simulink model "MPC_JUB27"  (R2020b)
settings: Solver=FixedStepDiscrete  StartTime=0.0  StopTime=StopTime  FixedStep=Ts  MaxStep=0.01  RelTol=1e-3
values from neighbouring files (symbols this model uses):
  dumax = [0.1; 1]    [CarregaDados.m]    (also in casadi_block_Control.m = evalin('base','dumax'))
  dumin = [0 ; 0]    [CarregaDados.m]    (also in casadi_block_Control.m = evalin('base','dumin'))
  f_buscaLimites_sym = evalin('base', 'f_buscaLimites_sym')    [casadi_block_Control.m]
  FreqAlvoIni = 55    [CarregaDados.m]
  Hc = 2    [CarregaDadosMPC.m]    (also in casadi_block_Control.m = evalin('base','Hc'))
  Hp = 5    [CarregaDadosMPC.m]    (also in casadi_block_Control.m = evalin('base','Hp'))
  LimiteProporcao = Ts/TempoESN    (= 641.025641026)    [CarregaDados.m]
  NumCasasDecimais = 1    [CarregaDados.m]
  PassoMPC = 3    [CarregaDadosMPC.m]
  Plano = readtable('PlanoAceleracaoErro.xlsx')    [CarregaDados.m]
  PMonAlvoIni = LimitaFaixa(PMonAlvoIni,FaixaPChegada)    [CarregaDados.m]
  Qu = diag([1  1])    [CarregaDadosMPC.m]    (also in casadi_block_Control.m = evalin('base','Qu'))
  Qy = diag([1  1])    [CarregaDadosMPC.m]    (also in casadi_block_Control.m = evalin('base','Qy'))
  R = [1  1]    [CarregaDadosMPC.m]    (also in casadi_block_Control.m = diag(repmat(R,1,Hc)))
  Rede_Processo = load('weightsESNx_TR300_TVaz0.8_RaioE0.1.mat')    [CarregaDados.m]
  SNR = 20    [CarregaDados.m]
  Ts = 10    [CarregaDados.m]
  UIni = repmat(UIni,Hc,1)    [casadi_block_Control.m]
  umax = [FreqMaxMin(1); PMonAlvoMaxMin(1)]    [CarregaDados.m]    (also in casadi_block_Control.m = evalin('base','umax'))
  umin = [FreqMaxMin(2); PMonAlvoMaxMin(2)]    [CarregaDados.m]    (also in casadi_block_Control.m = evalin('base','umin'))
  UsaPlano = 1    [CarregaDados.m]
  XIni = repmat(XIni,1+Hp,1)    [casadi_block_Control.m]
undefined symbols (not defined in the file or in its folder): awgn, BTP, Interpola, MatrizSimulador, MatrizSimuladorContas, TabelaIsometricas
libraries: simulink x1
settings Model: Creator=odilo  LastModifiedBy=leize
settings SolverCC: AlgebraicLoopSolver=LineSearch
settings DebuggingCC: InheritedTsInSrcMsg=none

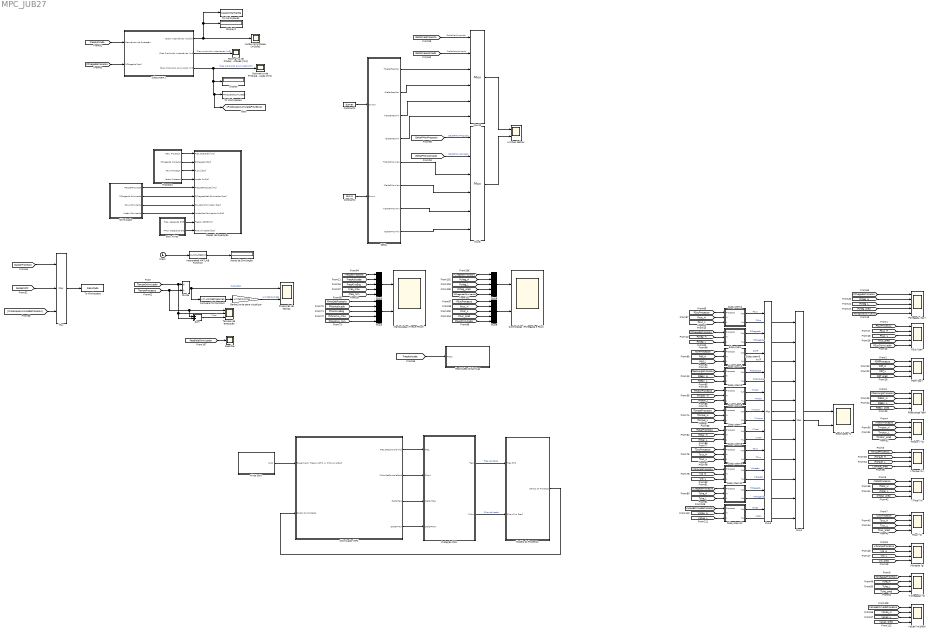
== system MPC_JUB27 ==
  Alvos ENG : Subsystem
  Clock : Clock
  Compare To Constant : simulink/Logic and Bit Operations/Compare To Constant  relop=<=  const=LimiteProporcao  OutDataTypeStr=boolean
  Constant1 : Constant  Value=dumax
  Constant2 : Constant  Value=dumin
  Controladas (PChegada e PSuc) : Scope  NumInputPorts=2
  Delta : Subsystem
  Display : Display
  Display3 : Display
  Divide : Product  Inputs=*/
  ENG. Alvos : Subsystem
  Estimativa de Produção Acumulada [m3] : Scope
  Estimativa de Produção instantânea [m3] : Scope
  Feasible : Scope
  GanhoLimite para visualizar : Gain  Gain=LimiteProporcao
  Horas de Simulação : Display
  I.Torque (A) : Scope  NumInputPorts=4
  I.Total (A) : Scope  NumInputPorts=4
  Interpreted MATLAB Function : MATLABFcn  MATLABFcn=round(u/3600,2)
  Limites DeltaU : Scope  NumInputPorts=2
  Manipuladas (Freq e PMon) : Scope  NumInputPorts=2
  Mapas de Operação : Subsystem  mask{PlotaMapas=1, HabilitaRastro=1, Tsim=MatrizSimulador, TsimContas=MatrizSimuladorContas, BTP=BTP, TabelaIsometricas=TabelaIsometricas, FreqIni=UIni(1), PChegadaIni=XIni(2), PSucIni=XIni(1), VazaoIni=XIni(11), FreqAlvoIni=FreqAlvoIni, PMonAlvoIni=PMonAlvoIni}
      mask prompts: PlotaMapas "Plotar Mapas (1/0)?"; HabilitaRastro "Habilita Rastro do Plot (1/0)?"; Tsim "Matriz do Simulador"; TsimContas "Matriz do Simulador para Limites"; BTP "Matriz BTP"; TabelaIsometricas "Tabela Curvas Isometricas"; FreqIni "Frequencia Inicial [Hz]"; PChegadaIni "PChegada Inicial [bar]"; PSucIni "PSuc Inicial [bar]"; VazaoIni "Vazao Inicial [m3/d]"; FreqAlvoIni "Frequencia ALVO Inicial [Hz]"; PMonAlvoIni "PChegada ALVO [bar]"
      mask DialogControl DescTextVar Prompt: MAPAS DE OPERAÇÃO
      mask DialogControl ParameterGroupVar Prompt: Tabelas Petrobras e configurações dos Mapas de Operação
      mask DialogControl ParameterGroupVar_copy Prompt: Dados do Processo
      mask DialogControl ParameterGroupVar_copy_copy_copy Prompt: Dados Engenharia (Alvos)
  Modelo do Processo : Subsystem  mask{ESN=Rede_Processo, YIni=XIni, UIni=UIni, SNR=SNR, NumCasasDecimais=NumCasasDecimais, MatrizSimulador=MatrizSimulador}
      mask prompts: ESN "Estruturada ESN"; YIni "Condicoes iniciais das variaveis"; UIni "Condicao Inicial das manipuladas (Freq e PMon)"; SNR "Relação Sinal Ruido aplicada"; NumCasasDecimais "Numero de casas decimais"; MatrizSimulador "Matriz do Simulador Petrobras"
  Mux : Mux  Inputs=3
  Mux{1..2,8..9} (4 alike) : Mux  Inputs=5
  Mux10 : Mux  Inputs=6
  Mux3 : Mux  Inputs=11
  Mux4 : Mux  Inputs=11
  Mux6 : Mux  Inputs=6
  Otimizador : Subsystem
  Otimizador MPC : Subsystem  mask{umax=umax, umin=umin, dumax=dumax, dumin=dumin, Hp=Hp, Hc=Hc, Qy=Qy, R=R, Qu=Qu, PassoMPC=PassoMPC}
      mask prompts: umax "Max valores para as manipuladas [Freq ;  PMonAlvo]"; umin "Min valores para as manipuladas [Freq ;  PMonAlvo]"; dumax "Max passo [Freq ;  PMonAlvo]"; dumin "Min passo [Freq ;  PMonAlvo]"; Hp "Horizonte de Predicao"; Hc "Horizonte de Controle"; Qy "Peso das Controladas [PSuc ; PChegada]"; R "Peso das Manipuladas [Freq ;  PMonAlvo]"; Qu "Peso dos alvos [Freq ;  PMonAlvo]"; PassoMPC "Passos para o controle atuar"
      mask DialogControl UserParameters Prompt: PARAMETROS DO USUARIO
      mask DialogControl ControlParameters Prompt: PARAMETROS DO CONTROLADOR
  PChegada (bar) : Scope  NumInputPorts=5
  PDescarga (bar) : Scope  NumInputPorts=4
  PDiff (bar) : Scope  NumInputPorts=4
  PSuc (bar) : Scope  NumInputPorts=5
  Processo : Subsystem
  Proporção de Tempo : Scope  NumInputPorts=2
  Proteção MPA : Subsystem  mask{DesabilitaMPA=0, DeltaUmax=dumax}
      mask prompts: DesabilitaMPA "Desabilita MPA"; DeltaUmax "Delta U Maximo (Freq e PMon)"
  Restrições % : Scope  NumInputPorts=2
  Restrições Dinâmicas : Subsystem
  Subsystem : Subsystem
  Subsystem1 : Subsystem  mask{MatrizSimulador=MatrizSimulador, DeltaT=Ts, QIni=XIni(11)}
      mask prompts: MatrizSimulador "Matriz do Simulador Petrobras"; DeltaT "Periodo de amostragem (s)"; QIni "Vazao Inicial (m3/dia)"
  Subsystem10 : Subsystem
  Subsystem12 : Subsystem
  Subsystem2 : Subsystem
  Subsystem3 : Subsystem
  Subsystem4 : Subsystem
  Subsystem5 : Subsystem
  Subsystem6 : Subsystem
  Subsystem7 : Subsystem
  Subsystem8 : Subsystem
  Subsystem9 : Subsystem
  Sum : Sum
  T.Chegada(°C) : Scope  NumInputPorts=4
  TMotor (°C) : Scope  NumInputPorts=4
  TSuc(°C) : Scope  NumInputPorts=4
  Tempos de execução : Scope  NumInputPorts=3
  To Workspace : ToWorkspace  VariableName=Resultado  SampleTime=-1
  To Workspace1 : ToWorkspace  VariableName=ProducaoAcumulada  SaveFormat=Timeseries  SampleTime=-1
  To Workspace2 : ToWorkspace  VariableName=VazaoInstantanea  SaveFormat=Timeseries  SampleTime=-1
  Vazão (m3/dia) : Scope  NumInputPorts=4
  Vazão Instantânea [m3/dia] : Scope
  Vibração (g) : Scope  NumInputPorts=4
  wires:
  [TempoProcesso] -> Sum/1, Tempos de execução/1, Divide/2
  [ITotalProcesso] -> I.Total (A)/1
  [TMotorProcesso] -> TMotor (°C)/1
  [VibracaoProcesso] -> Vibração (g)/1
  [TSucProcesso] -> TSuc(°C)/1
  [PDiffProcesso] -> PDiff (bar)/1
  [PDescargaProcesso] -> PDescarga (bar)/1
  [PSucProcesso] -> PSuc (bar)/1
  [Freq_max] -> Mux1/4
  [Freq_min] -> Mux1/5
  [FreqAlvoEng] -> Mux1/3
  [Psuc_H] -> PSuc (bar)/2
  [Psuc_L] -> PSuc (bar)/3
  [Pdif_H] -> PDiff (bar)/2
  [Pdif_L] -> PDiff (bar)/3
  [Pdif_pred] -> PDiff (bar)/4
  [Pdesc_H] -> PDescarga (bar)/2
  [Pdesc_L] -> PDescarga (bar)/3
  [Pdesc_pred] -> PDescarga (bar)/4
  [Tmotor_H] -> TMotor (°C)/2
  [Tmotor_L] -> TMotor (°C)/3
  [Tmotor_pred] -> TMotor (°C)/4
  [ITorqueProcesso] -> I.Torque (A)/1
  [ITorque_H] -> I.Torque (A)/2
  [ITorque_L] -> I.Torque (A)/3
  [Ctorque_pred] -> I.Torque (A)/4
  [ITotal_H] -> I.Total (A)/2
  [ITotal_L] -> I.Total (A)/3
  [CTotal_pred] -> I.Total (A)/4
  [Tsuc_H] -> TSuc(°C)/2
  [Tsuc_L] -> TSuc(°C)/3
  [Tsuc_pred] -> TSuc(°C)/4
  [Vib_H] -> Vibração (g)/2
  [Vib_L] -> Vibração (g)/3
  [Vib_pred] -> Vibração (g)/4
  [TChegadaProcesso] -> T.Chegada(°C)/1
  [Tche_H] -> T.Chegada(°C)/2
  [Tche_L] -> T.Chegada(°C)/3
  [Tche_pred] -> T.Chegada(°C)/4
  [SaidasMPC] -> Mux/2
  Mux/1 -> To Workspace/1
  [DadosProcesso] -> Mux/1
  Otimizador MPC/2(PMonSetControle[bar]) -> Proteção MPA/2(PMon.)
  [FreqAplicada] -> Mux1/2
  [Psuc_pred] -> PSuc (bar)/4
  [PSucOtimizador] -> PSuc (bar)/5
  [PChegadaProcesso] -> PChegada (bar)/1
  [Pcheg_H] -> PChegada (bar)/2
  [Pcheg_L] -> PChegada (bar)/3
  [Pcheg_pred] -> PChegada (bar)/4
  [PChegadaOtimizador] -> PChegada (bar)/5
  [TempoOtimizador] -> Sum/2, Tempos de execução/2, Divide/1
  Otimizador MPC/1(Freq.SetControle [Hz]) -> Proteção MPA/1(Freq.)
  [FreqAplicada] -> Subsystem1/1(Frequência de Operação)
  [PChegadaProcesso] -> Subsystem1/2(PChegada [bar])
  Subsystem1/2("Óleo Produzido Instantâneo (m3) ") -> Estimativa de Produção instantânea [m3]/1  "Óleo produzido Instantâneo (m3)"
  Subsystem1/3(Óleo Produzido Acumulado (m3)) -> [ProducaoAcumuladaProcesso], To Workspace1/1, Display/1, Estimativa de Produção Acumulada [m3]/1  "Óleo produzido acumulado(m3)"
  Subsystem1/1(Vazão Instantânea (m3/dia)) -> To Workspace2/1, Display3/1, Vazão Instantânea [m3/dia]/1
  Sum/1 -> Tempos de execução/3  "Total"
  Mux1/1 -> Manipuladas (Freq e PMon)/1
  [PMonAlvo_min] -> Mux2/5
  [PMonAlvo_max] -> Mux2/4
  [PMonAplicado] -> Mux2/2
  Mux2/1 -> Manipuladas (Freq e PMon)/2
  [PChegadaProcesso] -> Subsystem/1(Processo)
  [Pcheg_H] -> Subsystem/2(H)
  [Pcheg_L] -> Subsystem/3(L)
  [PSucProcesso] -> Subsystem2/1(Processo)
  [Psuc_H] -> Subsystem2/2(H)
  [Psuc_L] -> Subsystem2/3(L)
  [PDiffProcesso] -> Subsystem3/1(Processo)
  [Pdif_H] -> Subsystem3/2(H)
  [Pdif_L] -> Subsystem3/3(L)
  [PDescargaProcesso] -> Subsystem4/1(Processo)
  [Pdesc_H] -> Subsystem4/2(H)
  [Pdesc_L] -> Subsystem4/3(L)
  [Tmotor_L] -> Subsystem5/3(L)
  [Tmotor_H] -> Subsystem5/2(H)
  [TMotorProcesso] -> Subsystem5/1(Processo)
  [ITorqueProcesso] -> Subsystem6/1(Processo)
  [ITorque_H] -> Subsystem6/2(H)
  [ITorque_L] -> Subsystem6/3(L)
  [ITotalProcesso] -> Subsystem7/1(Processo)
  [ITotal_H] -> Subsystem7/2(H)
  [ITotal_L] -> Subsystem7/3(L)
  [TSucProcesso] -> Subsystem8/1(Processo)
  [Tsuc_H] -> Subsystem8/2(H)
  [Tsuc_L] -> Subsystem8/3(L)
  [VibracaoProcesso] -> Subsystem9/1(Processo)
  [Vib_H] -> Subsystem9/2(H)
  [Vib_L] -> Subsystem9/3(L)
  [TChegadaProcesso] -> Subsystem10/1(Processo)
  [Tche_H] -> Subsystem10/2(H)
  [Tche_L] -> Subsystem10/3(L)
  Mux3/1 -> Restrições %/1
  Mux4/1 -> Restrições %/2
  Subsystem/2(%L) -> Mux4/2  "PChegada"
  Subsystem2/2(%L) -> Mux4/1  "PSuc"
  Subsystem/1(%H) -> Mux3/2  "PChegada"
  Subsystem2/1(%H) -> Mux3/1  "PSuc"
  Subsystem3/1(%H) -> Mux3/3  "PDiff"
  Subsystem3/2(%L) -> Mux4/3  "PDiff"
  Subsystem4/1(%H) -> Mux3/4  "PDescarga"
  Subsystem4/2(%L) -> Mux4/4  "PDescarga"
  Subsystem5/2(%L) -> Mux4/5  "TMotor"
  Subsystem5/1(%H) -> Mux3/5  "TMotor"
  Subsystem6/2(%L) -> Mux4/6  "I.Torque"
  Subsystem6/1(%H) -> Mux3/6  "I.Torque"
  Subsystem7/2(%L) -> Mux4/7  "I.Total"
  Subsystem7/1(%H) -> Mux3/7  "I.Total"
  Subsystem8/2(%L) -> Mux4/8  "TSuc"
  Subsystem8/1(%H) -> Mux3/8  "TSuc"
  Subsystem9/2(%L) -> Mux4/9  "Vibração"
  Mux10/1 -> Limites DeltaU/1
  Constant1/1 -> Delta/1(dumax)
  Constant2/1 -> Delta/2(dumin)
  Delta/2(-DeltaFreqMax) -> Mux10/4
  Delta/3(+DeltaFreqMin) -> Mux10/5
  Delta/4(-DeltaFreqMin) -> Mux10/6
  Mux6/1 -> Limites DeltaU/2
  Clock/1 -> Interpreted MATLAB Function/1
  Interpreted MATLAB Function/1 -> Horas de Simulação/1
  [DeltaPMonProposto] -> Mux6/1  "DeltaPMonProposto"
  Delta/5(+DeltaPMonMax) -> Mux6/3
  Delta/6(-DeltaPMonMax) -> Mux6/4
  Delta/7(+DeltaPMonMin) -> Mux6/5
  Delta/8(-DeltaPMonMin) -> Mux6/6
  [PChegadaOtimizador] -> Mux8/5
  [Pcheg_pred] -> Mux8/4
  [Pcheg_L] -> Mux8/3
  [Pcheg_H] -> Mux8/2
  [PChegadaProcesso] -> Mux8/1
  [PSucOtimizador] -> Mux9/5
  [Psuc_pred] -> Mux9/4
  [Psuc_L] -> Mux9/3
  [Psuc_H] -> Mux9/2
  [PSucProcesso] -> Mux9/1
  Mux9/1 -> Controladas (PChegada e PSuc)/2
  Mux8/1 -> Controladas (PChegada e PSuc)/1
  [FeadibleOtimizador] -> Feasible/1
  Processo/1(Freq. Processo) -> Mapas de Operação/1(Freq.Operação [Hz])
  Processo/2(PChegada Processo) -> Mapas de Operação/2(PChegada [bar])
  Otimizador/2(PChegada Otimizador) -> Mapas de Operação/6(PChegadaSet Otimizador [bar])
  Otimizador/3(PSuc Otimizador) -> Mapas de Operação/7(PSucSet Otimizador [bar])
  ENG. Alvos/1(Freq. desejada ENG) -> Mapas de Operação/9(FreqAlvoENG[Hz])
  ENG. Alvos/2(PMon Desejada ENG) -> Mapas de Operação/10(PMonAlvoENG [bar])
  Processo/3(PSuc Processo) -> Mapas de Operação/3(P.Suc [bar])
  [DeltaFreqProposto] -> Mux10/1  "DeltaFreqProposto"
  [DeltaFreqAplicado] -> Mux10/2  "DeltaFreqAplicado"
  Delta/1(+DeltaFreqMax) -> Mux10/3
  [DeltaPMonAplicado] -> Mux6/2  "DeltaPMonAplicado"
  Proteção MPA/1(Freq) -> Modelo do Processo/1(Freq [Hz])  "Freq.Aplicada"
  Otimizador MPC/3(DeltaFreq) -> Proteção MPA/3(Delta Freq.)
  Otimizador MPC/4(DeltaPMon) -> Proteção MPA/4(DeltaPMon)
  Proteção MPA/2(PMon) -> Modelo do Processo/2(PMonAlvo [bar])  "PMonAplicada"
  [FreqSetProposta] -> Mux1/1
  [PMonSetProposto] -> Mux2/1
  Otimizador/1(FreqSetProposta) -> Mapas de Operação/5(FreqSetProposta [Hz])
  [PMonAlvoEng] -> Mux2/3
  [Vazao_L] -> Vazão (m3/dia)/3
  [Vazao_H] -> Vazão (m3/dia)/2
  [VazaoEstimadaProcesso] -> Vazão (m3/dia)/1
  [VazaoEstimadaProcesso] -> Subsystem12/1(Processo)
  [Vazao_H] -> Subsystem12/2(H)
  [Vazao_L] -> Subsystem12/3(L)
  Subsystem12/1(%H) -> Mux3/11  "Vazao"
  Subsystem12/2(%L) -> Mux4/11  "Vazao"
  Subsystem10/2(%L) -> Mux4/10  "TChegada"
  Subsystem9/1(%H) -> Mux3/9  "Vibração"
  Subsystem10/1(%H) -> Mux3/10  "TChegada"
  [Vazao_pred] -> Vazão (m3/dia)/4
  Modelo do Processo/1(Dados do Processo) -> Otimizador MPC/2(Dados do Processo)
  [ProducaoAcumuladaProcesso] -> Mux/3
  Divide/1 -> Proporção de Tempo/1, Compare To Constant/1  "Proporção"
  Compare To Constant/1 -> GanhoLimite para visualizar/1
  GanhoLimite para visualizar/1 -> Proporção de Tempo/2  "LimiteProporção"
  Processo/4(Vazão Processo) -> Mapas de Operação/4(Vazão [m3/d])
  Otimizador/4(Vazão Otimizador) -> Mapas de Operação/8(VazãoSet Otimizador [m3/d])
  Alvos ENG/1(Out1) -> Otimizador MPC/1(Engenharia: FreqAlvo[Hz]  e  PMonAlvo[bar])
  [FreqAplicada] -> Restrições Dinâmicas/1(Freq1)

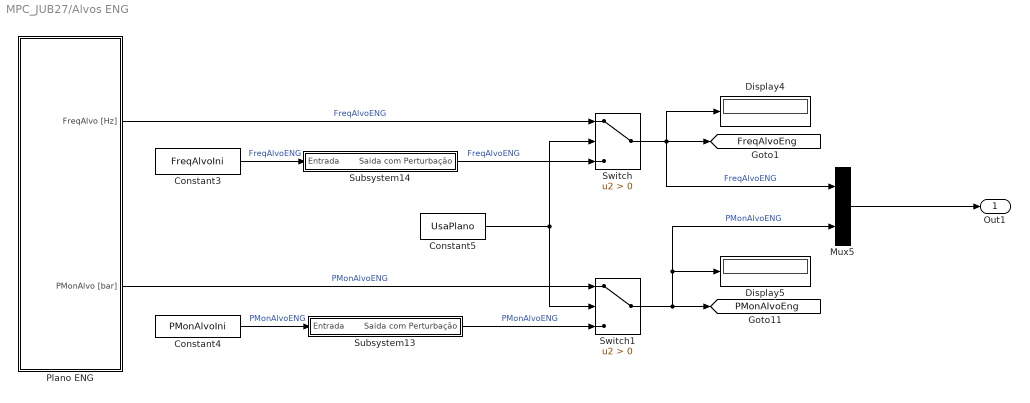
== system MPC_JUB27/Alvos ENG ==
  Constant3 : Constant  Value=FreqAlvoIni
  Constant4 : Constant  Value=PMonAlvoIni
  Constant5 : Constant  Value=UsaPlano
  Display4 : Display
  Display5 : Display
  Mux5 : Mux  Inputs=2
  Plano ENG : Subsystem  mask{Plano=Plano}
      mask prompts: Plano "Plano de Execucao"
      mask DialogControl DescGroupVar Prompt: TABELA COM PLANO DE EXECUCAO
  Subsystem13 : Subsystem  mask{TIni=1200, DeltaT=1.5*3600, ValorP=0}
      mask prompts: TIni "Tempo Inicio"; DeltaT "Duracao"; ValorP "Valor da Perturbacao"
  Subsystem14 : Subsystem  mask{TIni=1200, DeltaT=1.5*3600, ValorP=0}
      mask prompts: TIni "Tempo Inicio"; DeltaT "Duracao"; ValorP "Valor da Perturbacao"
  Switch : Switch  Criteria=u2 > Threshold
  Switch1 : Switch  Criteria=u2 > Threshold
  Out1 : Outport
  tag scope: FreqAlvoEng=global, PMonAlvoEng=global
  wires:
  Constant5/1 -> Switch1/2, Switch/2
  Subsystem14/1(Saida com Perturbação) -> Switch/3  "FreqAlvoENG"
  Switch1/1 -> Mux5/2, Display5/1, [PMonAlvoEng]  "PMonAlvoENG"
  Constant3/1 -> Subsystem14/1(Entrada)  "FreqAlvoENG"
  Constant4/1 -> Subsystem13/1(Entrada)  "PMonAlvoENG"
  Plano ENG/2(PMonAlvo [bar]) -> Switch1/1  "PMonAlvoENG"
  Switch/1 -> Mux5/1, [FreqAlvoEng], Display4/1  "FreqAlvoENG"
  Plano ENG/1(FreqAlvo [Hz]) -> Switch/1  "FreqAlvoENG"
  Subsystem13/1(Saida com Perturbação) -> Switch1/3  "PMonAlvoENG"
  Mux5/1 -> Out1/1

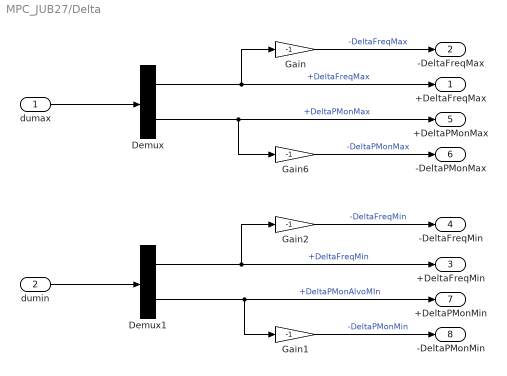
== system MPC_JUB27/Delta ==
  dumax : Inport
  dumin : Inport  Port=2
  Demux : Demux  Outputs=2
  Demux1 : Demux  Outputs=2
  Gain{,1..2,6} (4 alike) : Gain  Gain=-1
  +DeltaFreqMax : Outport
  -DeltaFreqMax : Outport  Port=2
  +DeltaFreqMin : Outport  Port=3
  -DeltaFreqMin : Outport  Port=4
  +DeltaPMonMax : Outport  Port=5
  -DeltaPMonMax : Outport  Port=6
  +DeltaPMonMin : Outport  Port=7
  -DeltaPMonMin : Outport  Port=8
  wires:
  Demux/1 -> Gain/1, +DeltaFreqMax/1  "+DeltaFreqMax"
  Demux1/2 -> Gain1/1, +DeltaPMonMin/1  "+DeltaPMonAlvoMIn"
  Demux/2 -> Gain6/1, +DeltaPMonMax/1  "+DeltaPMonMax"
  dumax/1 -> Demux/1
  dumin/1 -> Demux1/1
  Gain/1 -> -DeltaFreqMax/1  "-DeltaFreqMax"
  Gain2/1 -> -DeltaFreqMin/1  "-DeltaFreqMin"
  Demux1/1 -> Gain2/1, +DeltaFreqMin/1  "+DeltaFreqMin"
  Gain6/1 -> -DeltaPMonMax/1  "-DeltaPMonMax"
  Gain1/1 -> -DeltaPMonMin/1  "-DeltaPMonMin"

== system MPC_JUB27/ENG. Alvos ==
  Freq. desejada ENG : Outport
  PMon Desejada ENG : Outport  Port=2
  wires:
  [PMonAlvoEng] -> PMon Desejada ENG/1
  [FreqAlvoEng] -> Freq. desejada ENG/1

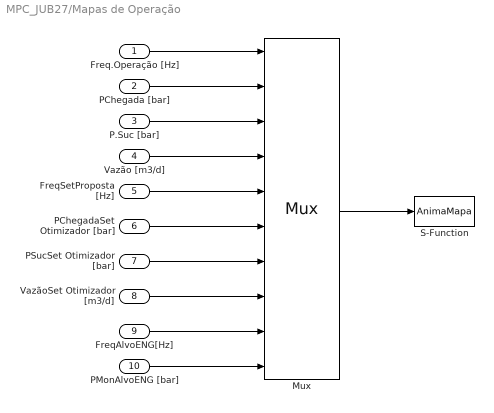
== system MPC_JUB27/Mapas de Operação ==
  Freq.Operação [Hz] : Inport
  PChegada [bar] : Inport  Port=2
  P.Suc [bar] : Inport  Port=3
  Vazão [m3/d] : Inport  Port=4
  FreqSetProposta [Hz] : Inport  Port=5
  PChegadaSet Otimizador [bar] : Inport  Port=6
  PSucSet Otimizador [bar] : Inport  Port=7
  VazãoSet Otimizador [m3/d] : Inport  Port=8
  FreqAlvoENG[Hz] : Inport  Port=9
  PMonAlvoENG [bar] : Inport  Port=10
  Mux : Mux  Inputs=10
  S-Function : S-Function  FunctionName=AnimaMapa  Parameters=PlotaMapas,Tsim,TsimContas,BTP,FreqIni, PChegadaIni,PSucIni,VazaoIni,FreqAlvoIni,PMonAlvoIni,HabilitaRastro,TabelaIsometricas  SFunctionDeploymentMode=off  EnableBusSupport=off
  wires:
  FreqSetProposta [Hz]/1 -> Mux/5
  PMonAlvoENG [bar]/1 -> Mux/10
  FreqAlvoENG[Hz]/1 -> Mux/9
  VazãoSet Otimizador [m3/d]/1 -> Mux/8
  PChegadaSet Otimizador [bar]/1 -> Mux/6
  Vazão [m3/d]/1 -> Mux/4
  PChegada [bar]/1 -> Mux/2
  Mux/1 -> S-Function/1
  Freq.Operação [Hz]/1 -> Mux/1
  P.Suc [bar]/1 -> Mux/3
  PSucSet Otimizador [bar]/1 -> Mux/7

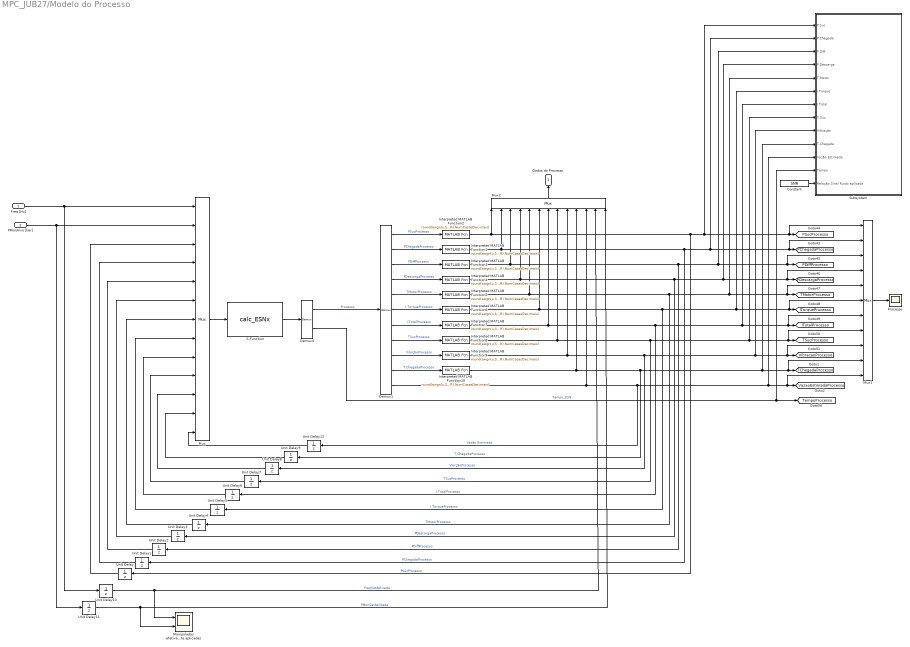
== system MPC_JUB27/Modelo do Processo ==
  Freq [Hz] : Inport
  PMonAlvo [bar] : Inport  Port=2
  Constant : Constant  Value=SNR
  Demux1 : Demux  Outputs=11
  Demux4 : Demux  Outputs=[ 11 1]
  Interpreted MATLAB Function{1..10} (10 alike) : MATLABFcn  MATLABFcn=round(awgn(u,SNR),NumCasasDecimais)
  Manipuladas efetivamente aplicadas : Scope  NumInputPorts=2
  Mux : Mux  Inputs=2+11
  Mux1 : Mux  Inputs=11
  Mux2 : Mux  Inputs=13
  Processo : Scope
  S-Function : S-Function  FunctionName=calc_ESNx  Parameters=ESN.data,YIni,MatrizSimulador  SFunctionDeploymentMode=off  EnableBusSupport=off
  Subsystem : Subsystem
  Unit Delay : UnitDelay  InitialCondition=YIni(1)  SampleTime=-1  HasFrameUpgradeWarning=on
  Unit Delay1 : UnitDelay  InitialCondition=YIni(2)  SampleTime=-1  HasFrameUpgradeWarning=on
  Unit Delay10 : UnitDelay  InitialCondition=UIni(1)  SampleTime=-1  HasFrameUpgradeWarning=on
  Unit Delay11 : UnitDelay  InitialCondition=UIni(2)  SampleTime=-1  HasFrameUpgradeWarning=on
  Unit Delay12 : UnitDelay  InitialCondition=YIni(11)  SampleTime=-1  HasFrameUpgradeWarning=on
  Unit Delay2 : UnitDelay  InitialCondition=YIni(3)  SampleTime=-1  HasFrameUpgradeWarning=on
  Unit Delay3 : UnitDelay  InitialCondition=YIni(4)  SampleTime=-1  HasFrameUpgradeWarning=on
  Unit Delay4 : UnitDelay  InitialCondition=YIni(5)  SampleTime=-1  HasFrameUpgradeWarning=on
  Unit Delay5 : UnitDelay  InitialCondition=YIni(6)  SampleTime=-1  HasFrameUpgradeWarning=on
  Unit Delay6 : UnitDelay  InitialCondition=YIni(7)  SampleTime=-1  HasFrameUpgradeWarning=on
  Unit Delay7 : UnitDelay  InitialCondition=YIni(8)  SampleTime=-1  HasFrameUpgradeWarning=on
  Unit Delay8 : UnitDelay  InitialCondition=YIni(9)  SampleTime=-1  HasFrameUpgradeWarning=on
  Unit Delay9 : UnitDelay  InitialCondition=YIni(10)  SampleTime=-1  HasFrameUpgradeWarning=on
  Dados do Processo : Outport
  tag scope: ITorqueProcesso=global, ITotalProcesso=global, PChegadaProcesso=global, PDescargaProcesso=global, PDiffProcesso=global, PSucProcesso=global, TChegadaProcesso=global, TMotorProcesso=global, TSucProcesso=global, TempoProcesso=global, VazaoEstimadaProcesso=global, VibracaoProcesso=global
  wires:
  Mux/1 -> S-Function/1
  PMonAlvo [bar]/1 -> Unit Delay11/1, Mux/2
  Freq [Hz]/1 -> Unit Delay10/1, Mux/1
  Unit Delay/1 -> Mux/3
  Unit Delay1/1 -> Mux/4
  Unit Delay2/1 -> Mux/5
  Unit Delay3/1 -> Mux/6
  Unit Delay4/1 -> Mux/7
  Unit Delay5/1 -> Mux/8
  Unit Delay6/1 -> Mux/9
  Unit Delay7/1 -> Mux/10
  Unit Delay8/1 -> Mux/11
  Unit Delay9/1 -> Mux/12
  S-Function/1 -> Demux4/1
  Demux1/4 -> Interpreted MATLAB Function4/1  "PDescargaProcesso"
  Demux1/3 -> Interpreted MATLAB Function3/1  "PDiffProcesso"
  Demux1/9 -> Interpreted MATLAB Function9/1  "VibrçãoProcesso"
  Demux1/7 -> Interpreted MATLAB Function7/1  "I.TotalProcesso"
  Demux1/10 -> Interpreted MATLAB Function10/1  "T,ChegadaProcesso"
  Demux4/2 -> Subsystem/12(Tempo), [TempoProcesso]  "Tempo_ESN"
  Mux1/1 -> Processo/1
  Interpreted MATLAB Function2/1 -> Unit Delay/1, Subsystem/1(P.Suc), Mux1/1, [PSucProcesso], Mux2/1  "PSucProcesso"
  Interpreted MATLAB Function1/1 -> Subsystem/2(P.Chegada), Mux1/2, [PChegadaProcesso], Unit Delay1/1, Mux2/2  "PChegadaProcesso"
  Interpreted MATLAB Function3/1 -> Subsystem/3(P.Diff), Mux1/3, [PDiffProcesso], Unit Delay2/1, Mux2/3  "PDiffProcesso"
  Interpreted MATLAB Function4/1 -> Subsystem/4(P.Descarga), Mux1/4, [PDescargaProcesso], Unit Delay3/1, Mux2/4  "PDescargaProcesso"
  Interpreted MATLAB Function5/1 -> Subsystem/5(T.Motor), Mux1/5, [TMotorProcesso], Unit Delay4/1, Mux2/5  "TMotorProcesso"
  Interpreted MATLAB Function6/1 -> Subsystem/6(I.Torque), Mux1/6, [ITorqueProcesso], Unit Delay5/1, Mux2/6  "I.TorqueProcesso"
  Interpreted MATLAB Function7/1 -> Subsystem/7(I.Total), Mux1/7, [ITotalProcesso], Unit Delay6/1, Mux2/7  "I.TotalProcesso"
  Interpreted MATLAB Function8/1 -> Subsystem/8(T.Suc), Mux1/8, [TSucProcesso], Unit Delay7/1, Mux2/8  "TSucProcesso"
  Interpreted MATLAB Function9/1 -> Subsystem/9(Vibração), Mux1/9, [VibracaoProcesso], Unit Delay8/1, Mux2/9  "VibrçãoProcesso"
  Interpreted MATLAB Function10/1 -> Unit Delay9/1, Mux1/10, [TChegadaProcesso], Subsystem/10(T.Chegada), Mux2/10  "T,ChegadaProcesso"
  Constant/1 -> Subsystem/13(Relação Sinal Ruido aplicada)
  Demux1/1 -> Interpreted MATLAB Function2/1  "PSucProcesso"
  Demux1/2 -> Interpreted MATLAB Function1/1  "PChegadaProcesso"
  Demux1/5 -> Interpreted MATLAB Function5/1  "TMotorProcesso"
  Demux1/6 -> Interpreted MATLAB Function6/1  "I.TorqueProcesso"
  Demux1/8 -> Interpreted MATLAB Function8/1  "TSucProcesso"
  Mux2/1 -> Dados do Processo/1
  Demux4/1 -> Demux1/1  "Processo"
  Unit Delay10/1 -> Mux2/12, Manipuladas efetivamente aplicadas/1  "FreqSetAplicada"
  Unit Delay11/1 -> Mux2/13, Manipuladas efetivamente aplicadas/2  "PMonSetAplicada"
  Demux1/11 -> Subsystem/11(Vazão Estimada), Mux1/11, [VazaoEstimadaProcesso], Unit Delay12/1, Mux2/11  "Vazão Estimada"
  Unit Delay12/1 -> Mux/13

== system MPC_JUB27/Otimizador ==
  Interpreted MATLAB Function : MATLABFcn  MATLABFcn=Interpola(u(1),u(2)*1.019716,MatrizSimulador,3)
  Mux : Mux  Inputs=2
  FreqSetProposta : Outport
  PChegada Otimizador : Outport  Port=2
  PSuc Otimizador : Outport  Port=3
  Vazão Otimizador : Outport  Port=4
  wires:
  [PSucOtimizador] -> PSuc Otimizador/1
  [PChegadaOtimizador] -> Mux/2, PChegada Otimizador/1
  [FreqSetProposta] -> Mux/1, FreqSetProposta/1
  Mux/1 -> Interpreted MATLAB Function/1
  Interpreted MATLAB Function/1 -> Vazão Otimizador/1

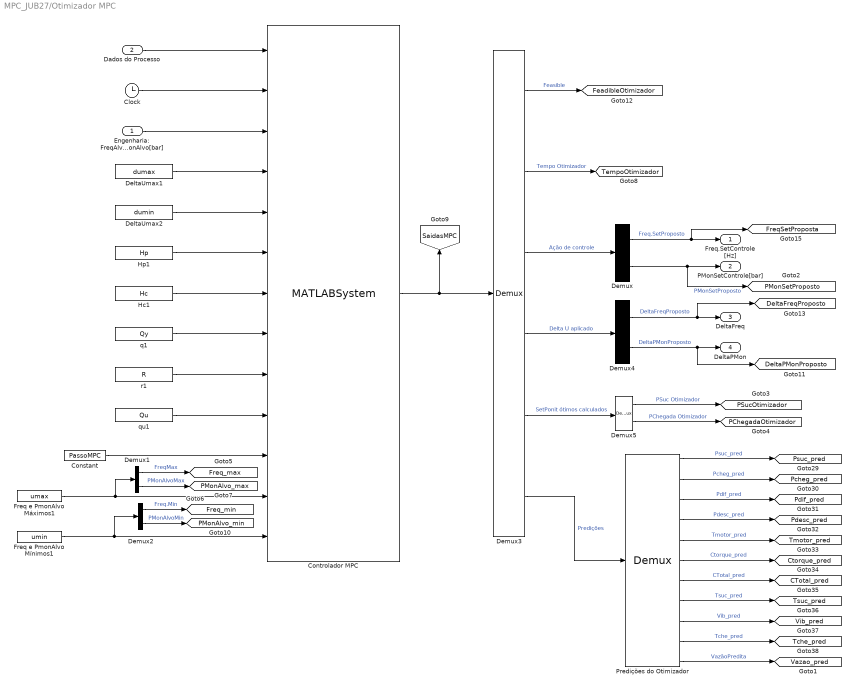
== system MPC_JUB27/Otimizador MPC ==
  Engenharia: FreqAlvo[Hz]  e  PMonAlvo[bar] : Inport
  Dados do Processo : Inport  Port=2
  Clock : Clock
  Constant : Constant  Value=PassoMPC
  Controlador MPC : MATLABSystem  System=casadi_block_Control  SimulateUsing=Interpreted execution
      mask Type: casadi_block_Control
      mask Display:
      | disp('casadi_block_Control');
      | port_label('input',1,'DadosProcesso');
      | port_label('input',2,'t');
      | port_label('input',3,'Alvos');
      | port_label('input',4,'dumax');
      | port_label('input',5,'dumin');
      | port_label('input',6,'Hp');
      | port_label('input',7,'Hc');
      | port_label('input',8,'Qy');
      | port_label('input',9,'R');
      | port_label('input',10,'Qu');
      | port_label('input',11,'PassoMPC');
      | port_label('input',12,'umax');
      | port_label('input',13,'umin');
      | port_label('output',1,'Saida');
  DeltaUmax1 : Constant  Value=dumax
  DeltaUmax2 : Constant  Value=dumin
  Demux{,1..2,4..5} (5 alike) : Demux  Outputs=2
  Demux3 : Demux  Outputs="[1  1  2  2  2  11]"
  Freq e PmonAlvo Máximos1 : Constant  Value=umax
  Freq e PmonAlvo Mínimos1 : Constant  Value=umin
  Hc1 : Constant  Value=Hc
  Hp1 : Constant  Value=Hp
  Predições do Otimizador : Demux  Outputs=11
  q1 : Constant  Value=Qy
  qu1 : Constant  Value=Qu
  r1 : Constant  Value=R
  Freq.SetControle [Hz] : Outport
  PMonSetControle[bar] : Outport  Port=2
  DeltaFreq : Outport  Port=3
  DeltaPMon : Outport  Port=4
  tag scope: CTotal_pred=global, Ctorque_pred=global, DeltaFreqProposto=global, DeltaPMonProposto=global, FeadibleOtimizador=global, FreqSetProposta=global, Freq_max=global, Freq_min=global, PChegadaOtimizador=global, PMonAlvo_max=global, PMonAlvo_min=global, PMonSetProposto=global, PSucOtimizador=global, Pcheg_pred=global, Pdesc_pred=global, Pdif_pred=global, Psuc_pred=global, SaidasMPC=global, Tche_pred=global, TempoOtimizador=global, Tmotor_pred=global, Tsuc_pred=global, Vazao_pred=global, Vib_pred=global
  wires:
  Dados do Processo/1 -> Controlador MPC/1
  Clock/1 -> Controlador MPC/2
  DeltaUmax1/1 -> Controlador MPC/4
  Hp1/1 -> Controlador MPC/6
  Hc1/1 -> Controlador MPC/7
  q1/1 -> Controlador MPC/8
  r1/1 -> Controlador MPC/9
  qu1/1 -> Controlador MPC/10
  Freq e PmonAlvo Máximos1/1 -> Demux1/1, Controlador MPC/12
  Freq e PmonAlvo Mínimos1/1 -> Demux2/1, Controlador MPC/13
  Predições do Otimizador/1 -> [Psuc_pred]  "Psuc_pred"
  Predições do Otimizador/2 -> [Pcheg_pred]  "Pcheg_pred"
  Predições do Otimizador/3 -> [Pdif_pred]  "Pdif_pred"
  Predições do Otimizador/4 -> [Pdesc_pred]  "Pdesc_pred"
  Predições do Otimizador/5 -> [Tmotor_pred]  "Tmotor_pred"
  Predições do Otimizador/6 -> [Ctorque_pred]  "Ctorque_pred"
  Predições do Otimizador/7 -> [CTotal_pred]  "CTotal_pred"
  Predições do Otimizador/8 -> [Tsuc_pred]  "Tsuc_pred"
  Predições do Otimizador/9 -> [Vib_pred]  "Vib_pred"
  Predições do Otimizador/10 -> [Tche_pred]  "Tche_pred"
  Demux1/2 -> [PMonAlvo_max]  "PMonAlvoMax"
  Demux1/1 -> [Freq_max]  "FreqMax"
  Engenharia: FreqAlvo[Hz]  e  PMonAlvo[bar]/1 -> Controlador MPC/3
  Demux2/1 -> [Freq_min]  "Freq.Min"
  Demux2/2 -> [PMonAlvo_min]  "PMonAlvoMin"
  Demux5/2 -> [PChegadaOtimizador]  "PChegada Otimizador"
  Demux3/2 -> [TempoOtimizador]  "Tempo Otimizador"
  Controlador MPC/1 -> [SaidasMPC], Demux3/1
  Demux3/1 -> [FeadibleOtimizador]  "Feasible"
  Demux3/6 -> Predições do Otimizador/1  "Predições"
  Demux3/5 -> Demux5/1  "SetPonit ótimos calculados"
  Constant/1 -> Controlador MPC/11
  DeltaUmax2/1 -> Controlador MPC/5
  Demux4/1 -> DeltaFreq/1, [DeltaFreqProposto]  "DeltaFreqProposto"
  Demux5/1 -> [PSucOtimizador]  "PSuc Otimizador"
  Demux3/4 -> Demux4/1  "Delta U aplicado"
  Demux3/3 -> Demux/1  "Ação de controle"
  Demux/1 -> [FreqSetProposta], Freq.SetControle [Hz]/1  "Freq.SetProposto"
  Demux/2 -> [PMonSetProposto], PMonSetControle[bar]/1  "PMonSetProposto"
  Demux4/2 -> [DeltaPMonProposto], DeltaPMon/1  "DeltaPMonProposto"
  Predições do Otimizador/11 -> [Vazao_pred]  "VazãoPredita"

== system MPC_JUB27/Processo ==
  Freq. Processo : Outport
  PChegada Processo : Outport  Port=2
  PSuc Processo : Outport  Port=3
  Vazão Processo : Outport  Port=4
  wires:
  [PSucProcesso] -> PSuc Processo/1
  [FreqAplicada] -> Freq. Processo/1
  [PChegadaProcesso] -> PChegada Processo/1
  [VazaoEstimadaProcesso] -> Vazão Processo/1

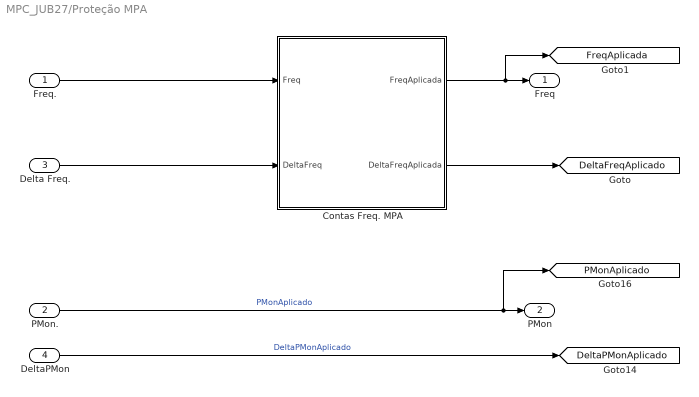
== system MPC_JUB27/Proteção MPA ==
  Freq. : Inport
  PMon. : Inport  Port=2
  Delta Freq. : Inport  Port=3
  DeltaPMon : Inport  Port=4
  Contas Freq. MPA : Subsystem
  Freq : Outport
  PMon : Outport  Port=2
  tag scope: DeltaFreqAplicado=global, DeltaPMonAplicado=global, FreqAplicada=global, PMonAplicado=global
  wires:
  Freq./1 -> Contas Freq. MPA/1(Freq)
  DeltaPMon/1 -> [DeltaPMonAplicado]  "DeltaPMonAplicado"
  PMon./1 -> [PMonAplicado], PMon/1  "PMonAplicado"
  Contas Freq. MPA/1(FreqAplicada) -> Freq/1, [FreqAplicada]
  Delta Freq./1 -> Contas Freq. MPA/2(DeltaFreq)
  Contas Freq. MPA/2(DeltaFreqAplicada) -> [DeltaFreqAplicado]

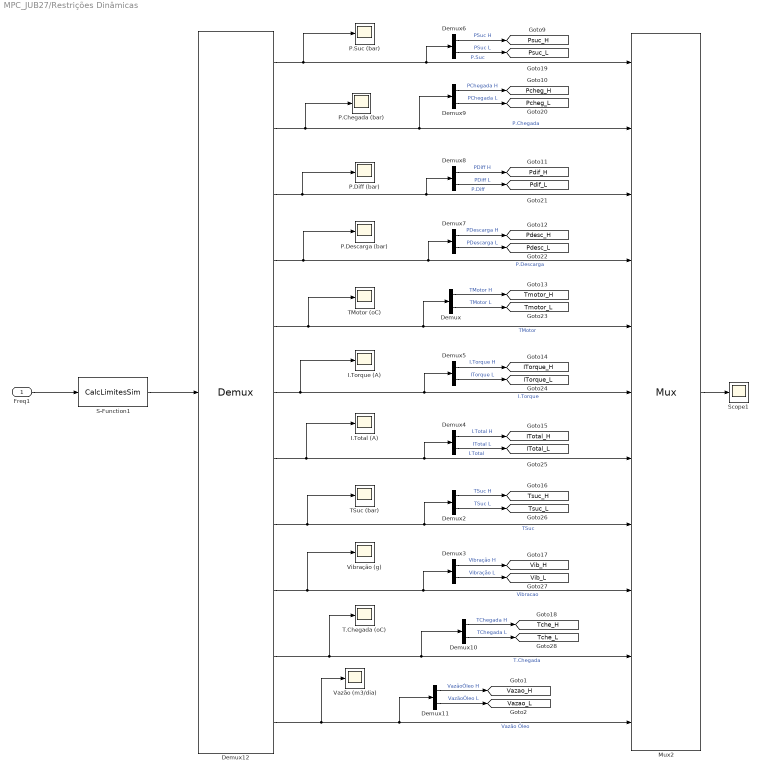
== system MPC_JUB27/Restrições Dinâmicas ==
  Freq1 : Inport
  Demux{,2..11} (11 alike) : Demux  Outputs=2
  Demux12 : Demux  Outputs=[ 2 2 2 2 2 2 2 2 2 2 2]
  I.Torque (A) : Scope
  I.Total (A) : Scope
  Mux2 : Mux  Inputs=[ 2 2 2 2 2 2 2 2 2 2 2]
  P.Chegada (bar) : Scope
  P.Descarga (bar) : Scope
  P.Diff (bar) : Scope
  P.Suc (bar) : Scope
  S-Function1 : S-Function  FunctionName=CalcLimitesSim  Parameters=UIni(1),f_buscaLimites_sym  SFunctionDeploymentMode=off  EnableBusSupport=off
  Scope1 : Scope
  T.Chegada (oC) : Scope
  TMotor (oC) : Scope
  TSuc (bar) : Scope
  Vazão (m3/dia) : Scope
  Vibração (g) : Scope
  tag scope: ITorque_H=global, ITorque_L=global, ITotal_H=global, ITotal_L=global, Pcheg_H=global, Pcheg_L=global, Pdesc_H=global, Pdesc_L=global, Pdif_H=global, Pdif_L=global, Psuc_H=global, Psuc_L=global, Tche_H=global, Tche_L=global, Tmotor_H=global, Tmotor_L=global, Tsuc_H=global, Tsuc_L=global, Vazao_H=global, Vazao_L=global, Vib_H=global, Vib_L=global
  wires:
  Demux12/9 -> Vibração (g)/1, Demux3/1, Mux2/9  "Vibracao"
  Demux12/4 -> P.Descarga (bar)/1, Demux7/1, Mux2/4  "P.Descarga"
  Demux12/10 -> T.Chegada (oC)/1, Demux10/1, Mux2/10  "T.Chegada"
  Demux12/1 -> P.Suc (bar)/1, Mux2/1, Demux6/1  "P.Suc"
  Demux12/2 -> P.Chegada (bar)/1, Demux9/1, Mux2/2  "P.Chegada"
  Demux12/3 -> P.Diff (bar)/1, Mux2/3, Demux8/1  "P.Diff"
  Demux12/5 -> TMotor (oC)/1, Demux/1, Mux2/5  "TMotor"
  Demux12/8 -> TSuc (bar)/1, Demux2/1, Mux2/8  "TSuc"
  Demux12/6 -> I.Torque (A)/1, Demux5/1, Mux2/6  "I.Torque"
  Demux12/7 -> I.Total (A)/1, Demux4/1, Mux2/7  "I.Total"
  Demux/2 -> [Tmotor_L]  "TMotor L"
  Demux/1 -> [Tmotor_H]  "TMotor H"
  Demux6/1 -> [Psuc_H]  "PSuc H"
  Demux9/1 -> [Pcheg_H]  "PChegada H"
  Demux8/1 -> [Pdif_H]  "PDiff H"
  Demux7/1 -> [Pdesc_H]  "PDescarga H"
  Demux5/1 -> [ITorque_H]  "I.Torque H"
  Demux4/1 -> [ITotal_H]  "I.Total H"
  Demux2/1 -> [Tsuc_H]  "TSuc H"
  Demux3/1 -> [Vib_H]  "Vibração H"
  Demux10/1 -> [Tche_H]  "TChegada H"
  Demux6/2 -> [Psuc_L]  "PSuc L"
  Demux9/2 -> [Pcheg_L]  "PChegada L"
  Demux8/2 -> [Pdif_L]  "PDiff L"
  Demux7/2 -> [Pdesc_L]  "PDescarga L"
  Demux4/2 -> [ITotal_L]  "ITotal L"
  Demux2/2 -> [Tsuc_L]  "TSuc L"
  Demux3/2 -> [Vib_L]  "Vibração L"
  Demux10/2 -> [Tche_L]  "TChegada L"
  Demux5/2 -> [ITorque_L]  "ITorque L"
  Demux12/11 -> Demux11/1, Mux2/11, Vazão (m3/dia)/1  "Vazão Óleo"
  Demux11/2 -> [Vazao_L]  "VazãoÓleo L"
  Demux11/1 -> [Vazao_H]  "VazãoÓleo H"
  S-Function1/1 -> Demux12/1
  Freq1/1 -> S-Function1/1
  Mux2/1 -> Scope1/1

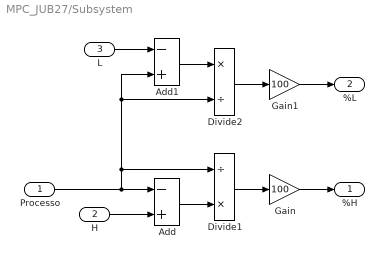
== system MPC_JUB27/Subsystem ==
  Processo : Inport
  H : Inport  Port=2
  L : Inport  Port=3
  Add : Sum  Inputs=-+
  Add1 : Sum  Inputs=-+
  Divide1 : Product  Inputs=/*
  Divide2 : Product  Inputs=*/
  Gain : Gain  Gain=100
  Gain1 : Gain  Gain=100
  %H : Outport
  %L : Outport  Port=2
  wires:
  H/1 -> Add/2
  Processo/1 -> Add/1, Divide1/1, Divide2/2, Add1/2
  Divide1/1 -> Gain/1
  Gain/1 -> %H/1
  L/1 -> Add1/1
  Gain1/1 -> %L/1
  Divide2/1 -> Gain1/1
  Add1/1 -> Divide2/1
  Add/1 -> Divide1/2

== system MPC_JUB27/Subsystem1 ==
  Frequência de Operação : Inport
  PChegada [bar] : Inport  Port=2
  Demux : Demux  Outputs=3
  Mux : Mux  Inputs=2
  S-function1 : S-Function  FunctionName=CalcVazao  Parameters=MatrizSimulador,DeltaT,QIni  SFunctionDeploymentMode=off  EnableBusSupport=off
  Vazão Instantânea (m3/dia) : Outport
  "Óleo Produzido Instantâneo (m3) " : Outport  Port=2
  Óleo Produzido Acumulado (m3) : Outport  Port=3
  wires:
  PChegada [bar]/1 -> Mux/2
  Frequência de Operação/1 -> Mux/1
  Mux/1 -> S-function1/1
  S-function1/1 -> Demux/1
  Demux/2 -> "Óleo Produzido Instantâneo (m3) "/1
  Demux/3 -> Óleo Produzido Acumulado (m3)/1
  Demux/1 -> Vazão Instantânea (m3/dia)/1

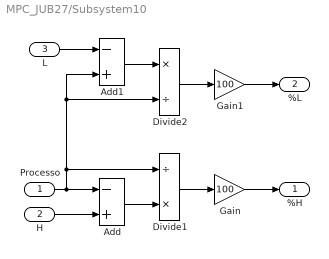
== system MPC_JUB27/Subsystem10 ==
  Processo : Inport
  H : Inport  Port=2
  L : Inport  Port=3
  Add : Sum  Inputs=-+
  Add1 : Sum  Inputs=-+
  Divide1 : Product  Inputs=/*
  Divide2 : Product  Inputs=*/
  Gain : Gain  Gain=100
  Gain1 : Gain  Gain=100
  %H : Outport
  %L : Outport  Port=2
  wires:
  Add/1 -> Divide1/2
  Add1/1 -> Divide2/1
  Divide2/1 -> Gain1/1
  Gain1/1 -> %L/1
  L/1 -> Add1/1
  Gain/1 -> %H/1
  Divide1/1 -> Gain/1
  Processo/1 -> Add1/2, Divide2/2, Divide1/1, Add/1
  H/1 -> Add/2

== system MPC_JUB27/Subsystem12 ==
  Processo : Inport
  H : Inport  Port=2
  L : Inport  Port=3
  Add : Sum  Inputs=-+
  Add1 : Sum  Inputs=-+
  Divide1 : Product  Inputs=/*
  Divide2 : Product  Inputs=*/
  Gain : Gain  Gain=100
  Gain1 : Gain  Gain=100
  %H : Outport
  %L : Outport  Port=2
  wires:
  H/1 -> Add/2
  Processo/1 -> Add/1, Divide1/1, Divide2/2, Add1/2
  Divide1/1 -> Gain/1
  Gain/1 -> %H/1
  L/1 -> Add1/1
  Gain1/1 -> %L/1
  Divide2/1 -> Gain1/1
  Add1/1 -> Divide2/1
  Add/1 -> Divide1/2

== system MPC_JUB27/Subsystem2 ==
  Processo : Inport
  H : Inport  Port=2
  L : Inport  Port=3
  Add : Sum  Inputs=-+
  Add1 : Sum  Inputs=-+
  Divide1 : Product  Inputs=/*
  Divide2 : Product  Inputs=*/
  Gain : Gain  Gain=100
  Gain1 : Gain  Gain=100
  %H : Outport
  %L : Outport  Port=2
  wires:
  Add/1 -> Divide1/2
  Add1/1 -> Divide2/1
  Divide2/1 -> Gain1/1
  Gain1/1 -> %L/1
  L/1 -> Add1/1
  Gain/1 -> %H/1
  Divide1/1 -> Gain/1
  Processo/1 -> Add1/2, Divide2/2, Divide1/1, Add/1
  H/1 -> Add/2

== system MPC_JUB27/Subsystem3 ==
  Processo : Inport
  H : Inport  Port=2
  L : Inport  Port=3
  Add : Sum  Inputs=-+
  Add1 : Sum  Inputs=-+
  Divide1 : Product  Inputs=/*
  Divide2 : Product  Inputs=*/
  Gain : Gain  Gain=100
  Gain1 : Gain  Gain=100
  %H : Outport
  %L : Outport  Port=2
  wires:
  H/1 -> Add/2
  Processo/1 -> Add/1, Divide1/1, Divide2/2, Add1/2
  Divide1/1 -> Gain/1
  Gain/1 -> %H/1
  L/1 -> Add1/1
  Gain1/1 -> %L/1
  Divide2/1 -> Gain1/1
  Add1/1 -> Divide2/1
  Add/1 -> Divide1/2

== system MPC_JUB27/Subsystem4 ==
  Processo : Inport
  H : Inport  Port=2
  L : Inport  Port=3
  Add : Sum  Inputs=-+
  Add1 : Sum  Inputs=-+
  Divide1 : Product  Inputs=/*
  Divide2 : Product  Inputs=*/
  Gain : Gain  Gain=100
  Gain1 : Gain  Gain=100
  %H : Outport
  %L : Outport  Port=2
  wires:
  Add/1 -> Divide1/2
  Add1/1 -> Divide2/1
  Divide2/1 -> Gain1/1
  Gain1/1 -> %L/1
  L/1 -> Add1/1
  Gain/1 -> %H/1
  Divide1/1 -> Gain/1
  Processo/1 -> Add1/2, Divide2/2, Divide1/1, Add/1
  H/1 -> Add/2

== system MPC_JUB27/Subsystem5 ==
  Processo : Inport
  H : Inport  Port=2
  L : Inport  Port=3
  Add : Sum  Inputs=-+
  Add1 : Sum  Inputs=-+
  Divide1 : Product  Inputs=/*
  Divide2 : Product  Inputs=*/
  Gain : Gain  Gain=100
  Gain1 : Gain  Gain=100
  %H : Outport
  %L : Outport  Port=2
  wires:
  H/1 -> Add/2
  Processo/1 -> Add/1, Divide1/1, Divide2/2, Add1/2
  Divide1/1 -> Gain/1
  Gain/1 -> %H/1
  L/1 -> Add1/1
  Gain1/1 -> %L/1
  Divide2/1 -> Gain1/1
  Add1/1 -> Divide2/1
  Add/1 -> Divide1/2

== system MPC_JUB27/Subsystem6 ==
  Processo : Inport
  H : Inport  Port=2
  L : Inport  Port=3
  Add : Sum  Inputs=-+
  Add1 : Sum  Inputs=-+
  Divide1 : Product  Inputs=/*
  Divide2 : Product  Inputs=*/
  Gain : Gain  Gain=100
  Gain1 : Gain  Gain=100
  %H : Outport
  %L : Outport  Port=2
  wires:
  Add/1 -> Divide1/2
  Add1/1 -> Divide2/1
  Divide2/1 -> Gain1/1
  Gain1/1 -> %L/1
  L/1 -> Add1/1
  Gain/1 -> %H/1
  Divide1/1 -> Gain/1
  Processo/1 -> Add1/2, Divide2/2, Divide1/1, Add/1
  H/1 -> Add/2

== system MPC_JUB27/Subsystem7 ==
  Processo : Inport
  H : Inport  Port=2
  L : Inport  Port=3
  Add : Sum  Inputs=-+
  Add1 : Sum  Inputs=-+
  Divide1 : Product  Inputs=/*
  Divide2 : Product  Inputs=*/
  Gain : Gain  Gain=100
  Gain1 : Gain  Gain=100
  %H : Outport
  %L : Outport  Port=2
  wires:
  H/1 -> Add/2
  Processo/1 -> Add/1, Divide1/1, Divide2/2, Add1/2
  Divide1/1 -> Gain/1
  Gain/1 -> %H/1
  L/1 -> Add1/1
  Gain1/1 -> %L/1
  Divide2/1 -> Gain1/1
  Add1/1 -> Divide2/1
  Add/1 -> Divide1/2

== system MPC_JUB27/Subsystem8 ==
  Processo : Inport
  H : Inport  Port=2
  L : Inport  Port=3
  Add : Sum  Inputs=-+
  Add1 : Sum  Inputs=-+
  Divide1 : Product  Inputs=/*
  Divide2 : Product  Inputs=*/
  Gain : Gain  Gain=100
  Gain1 : Gain  Gain=100
  %H : Outport
  %L : Outport  Port=2
  wires:
  Add/1 -> Divide1/2
  Add1/1 -> Divide2/1
  Divide2/1 -> Gain1/1
  Gain1/1 -> %L/1
  L/1 -> Add1/1
  Gain/1 -> %H/1
  Divide1/1 -> Gain/1
  Processo/1 -> Add1/2, Divide2/2, Divide1/1, Add/1
  H/1 -> Add/2

== system MPC_JUB27/Subsystem9 ==
  Processo : Inport
  H : Inport  Port=2
  L : Inport  Port=3
  Add : Sum  Inputs=-+
  Add1 : Sum  Inputs=-+
  Divide1 : Product  Inputs=/*
  Divide2 : Product  Inputs=*/
  Gain : Gain  Gain=100
  Gain1 : Gain  Gain=100
  %H : Outport
  %L : Outport  Port=2
  wires:
  H/1 -> Add/2
  Processo/1 -> Add/1, Divide1/1, Divide2/2, Add1/2
  Divide1/1 -> Gain/1
  Gain/1 -> %H/1
  L/1 -> Add1/1
  Gain1/1 -> %L/1
  Divide2/1 -> Gain1/1
  Add1/1 -> Divide2/1
  Add/1 -> Divide1/2

== system MPC_JUB27/Alvos ENG/Plano ENG ==
  Demux : Demux  Outputs=2
  S-Function : S-Function  FunctionName=ExecutaPlano  Parameters=Plano  SFunctionDeploymentMode=off  EnableBusSupport=off
  FreqAlvo [Hz] : Outport
  PMonAlvo [bar] : Outport  Port=2
  wires:
  S-Function/1 -> Demux/1
  Demux/1 -> FreqAlvo [Hz]/1  "Freq"
  Demux/2 -> PMonAlvo [bar]/1  "PMonAlvo"

== system MPC_JUB27/Alvos ENG/Subsystem13 ==
  Entrada : Inport
  Add : Sum  Inputs=++-
  Delay : Delay  DelayLength=DeltaT/Ts
  Perturbação1 : Step  Time=TIni  After=ValorP  SampleTime=0
  Saida com Perturbação : Outport
  wires:
  Entrada/1 -> Add/2
  Delay/1 -> Add/3
  Add/1 -> Saida com Perturbação/1
  Perturbação1/1 -> Add/1, Delay/1

== system MPC_JUB27/Alvos ENG/Subsystem14 ==
  Entrada : Inport
  Add : Sum  Inputs=++-
  Delay : Delay  DelayLength=DeltaT/Ts
  Perturbação1 : Step  Time=TIni  After=ValorP  SampleTime=0
  Saida com Perturbação : Outport
  wires:
  Perturbação1/1 -> Delay/1, Add/1
  Add/1 -> Saida com Perturbação/1
  Delay/1 -> Add/3
  Entrada/1 -> Add/2

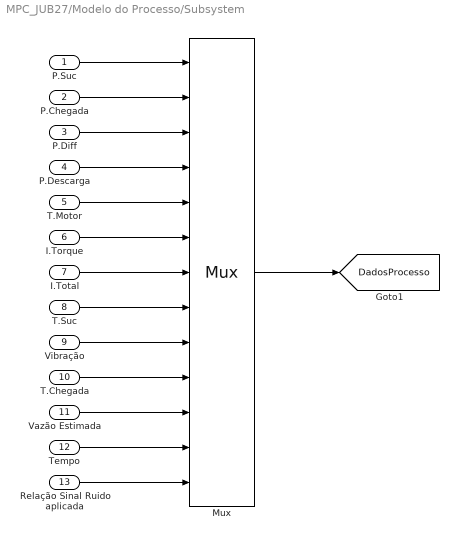
== system MPC_JUB27/Modelo do Processo/Subsystem ==
  P.Suc : Inport
  P.Chegada : Inport  Port=2
  P.Diff : Inport  Port=3
  P.Descarga : Inport  Port=4
  T.Motor : Inport  Port=5
  I.Torque : Inport  Port=6
  I.Total : Inport  Port=7
  T.Suc : Inport  Port=8
  Vibração : Inport  Port=9
  T.Chegada : Inport  Port=10
  Vazão Estimada : Inport  Port=11
  Tempo : Inport  Port=12
  Relação Sinal Ruido aplicada : Inport  Port=13
  Mux : Mux  Inputs=13
  tag scope: DadosProcesso=global
  wires:
  P.Suc/1 -> Mux/1
  P.Chegada/1 -> Mux/2
  T.Motor/1 -> Mux/5
  I.Torque/1 -> Mux/6
  T.Suc/1 -> Mux/8
  P.Diff/1 -> Mux/3
  I.Total/1 -> Mux/7
  P.Descarga/1 -> Mux/4
  Mux/1 -> [DadosProcesso]
  T.Chegada/1 -> Mux/10
  Vibração/1 -> Mux/9
  Relação Sinal Ruido aplicada/1 -> Mux/13
  Vazão Estimada/1 -> Mux/11
  Tempo/1 -> Mux/12

== system MPC_JUB27/Proteção MPA/Contas Freq. MPA ==
  Freq : Inport
  DeltaFreq : Inport  Port=2
  Constant : Constant  Value=DesabilitaMPA
  Inibe alteração da Freq nos limite de 1Hz a cada 7,5min : Subsystem
  Switch : Switch  Criteria=u2 > Threshold
  Switch1 : Switch  Criteria=u2 > Threshold
  FreqAplicada : Outport
  DeltaFreqAplicada : Outport  Port=2
  wires:
  DeltaFreq/1 -> Inibe alteração da Freq nos limite de 1Hz a cada 7,5min/2(DeltaFreq (k)), Switch1/1
  Constant/1 -> Switch1/2, Switch/2
  Switch1/1 -> DeltaFreqAplicada/1  "DeltaFreqAplicada"
  Freq/1 -> Switch/1, Inibe alteração da Freq nos limite de 1Hz a cada 7,5min/1(Freq)
  Inibe alteração da Freq nos limite de 1Hz a cada 7,5min/1(FreqAplicada) -> Switch/3
  Inibe alteração da Freq nos limite de 1Hz a cada 7,5min/2(DeltaFreqAplicado) -> Switch1/3
  Switch/1 -> FreqAplicada/1  "FreqAplicada"

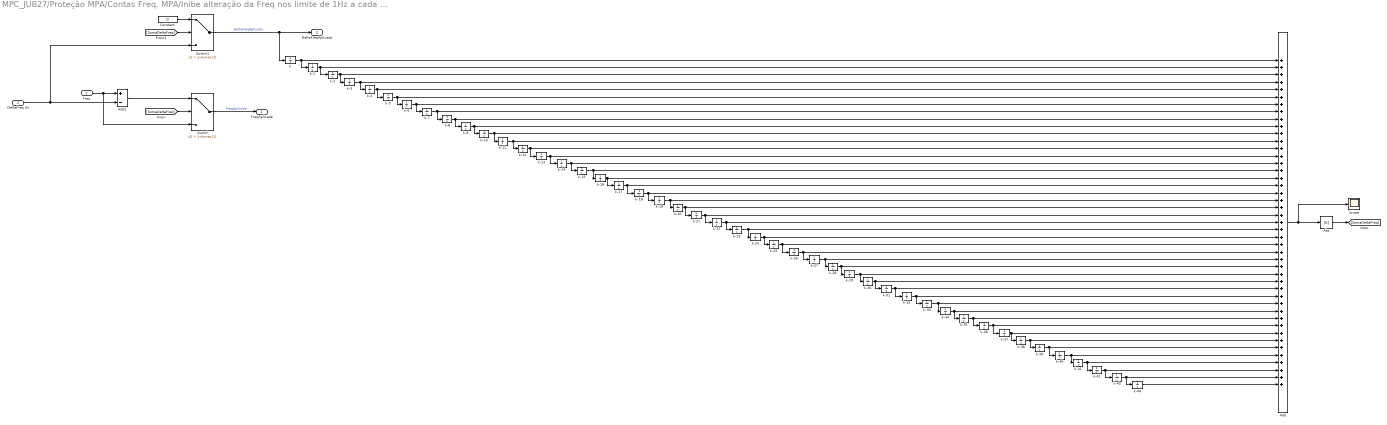
== system MPC_JUB27/Proteção MPA/Contas Freq. MPA/Inibe alteração da Freq nos limite de 1Hz a cada 7,5min ==
  Freq : Inport
  DeltaFreq (k) : Inport  Port=2
  Abs : Abs
  Add : Sum  Inputs=+++++++++++++++++++++++++++++++++++++++++++++
  Add1 : Sum  Inputs=+-
  Constant : Constant  Value=0
  Scope : Scope
  Switch : Switch  Criteria=u2 > Threshold  Threshold=1-dumax(1)
  Switch1 : Switch  Criteria=u2 > Threshold  Threshold=1-dumax(1)
  k : UnitDelay  SampleTime=-1  HasFrameUpgradeWarning=on
  k-{1..44} (44 alike) : UnitDelay  SampleTime=-1  HasFrameUpgradeWarning=on
  FreqAplicada : Outport
  DeltaFreqAplicado : Outport  Port=2
  wires:
  DeltaFreq (k)/1 -> Switch1/3, Add1/2
  k-1/1 -> k-2/1, Add/2
  k-2/1 -> Add/3, k-3/1
  k-3/1 -> Add/4, k-4/1
  k-4/1 -> Add/5, k-5/1
  k-5/1 -> Add/6, k-6/1
  k-7/1 -> Add/8, k-8/1
  k-9/1 -> Add/10, k-10/1
  k-6/1 -> Add/7, k-7/1
  k-13/1 -> Add/14, k-14/1
  k-10/1 -> Add/11, k-11/1
  [SomaDeltaFreq] -> Switch/2
  [SomaDeltaFreq] -> Switch1/2
  Switch/1 -> FreqAplicada/1  "FreqAplicada"
  Switch1/1 -> k/1, DeltaFreqAplicado/1  "DeltaFreqAplicado"
  Constant/1 -> Switch1/1
  Freq/1 -> Switch/3, Add1/1
  Add1/1 -> Switch/1
  k/1 -> k-1/1, Add/1
  k-8/1 -> Add/9, k-9/1
  k-11/1 -> Add/12, k-12/1
  k-12/1 -> Add/13, k-13/1
  k-14/1 -> k-15/1, Add/15
  k-15/1 -> k-16/1, Add/16
  k-19/1 -> Add/20, k-20/1
  k-18/1 -> Add/19, k-19/1
  k-16/1 -> k-17/1, Add/17
  k-17/1 -> Add/18, k-18/1
  k-21/1 -> Add/22, k-22/1
  k-20/1 -> k-21/1, Add/21
  k-22/1 -> Add/23, k-23/1
  k-23/1 -> Add/24, k-24/1
  Add/1 -> Scope/1, Abs/1
  k-28/1 -> k-29/1, Add/29
  k-27/1 -> Add/28, k-28/1
  k-26/1 -> Add/27, k-27/1
  k-24/1 -> k-25/1, Add/25
  k-25/1 -> Add/26, k-26/1
  k-35/1 -> Add/36, k-36/1
  k-34/1 -> Add/35, k-35/1
  k-36/1 -> Add/37, k-37/1
  k-37/1 -> Add/38, k-38/1
  k-38/1 -> k-39/1, Add/39
  k-33/1 -> Add/34, k-34/1
  k-32/1 -> Add/33, k-33/1
  k-30/1 -> Add/31, k-31/1
  k-31/1 -> Add/32, k-32/1
  k-29/1 -> k-30/1, Add/30
  k-39/1 -> k-40/1, Add/40
  k-40/1 -> Add/41, k-41/1
  k-44/1 -> Add/45
  k-43/1 -> Add/44, k-44/1
  k-41/1 -> Add/42, k-42/1
  k-42/1 -> Add/43, k-43/1
  Abs/1 -> [SomaDeltaFreq]
